simulink model "airbeats"  (R2022a)
settings: Solver=VariableStepAuto  StartTime=0.0  StopTime=10.0  RelTol=1e-3
settings Model: Creator=shobh  LastModifiedBy=shobh

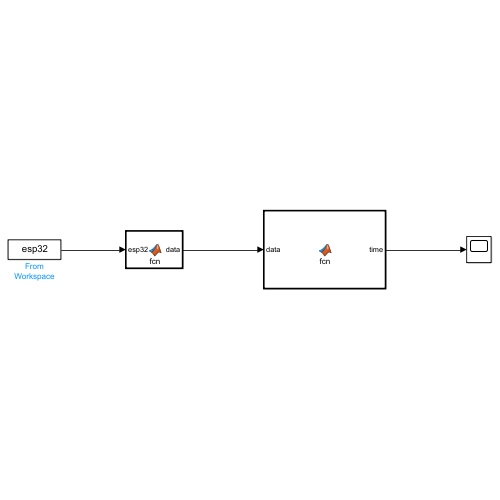
[thumbnail: Simulink's stored preview of the top-level diagram]
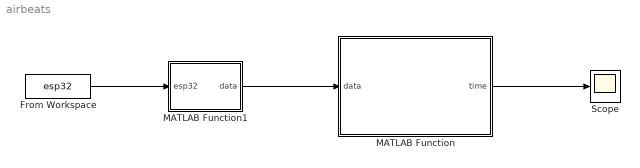
== system airbeats ==
  From Workspace : FromWorkspace  VariableName=esp32
  MATLAB Function : MATLAB Function  TreatAsAtomicUnit=on
  MATLAB Function1 : MATLAB Function  TreatAsAtomicUnit=on
  Scope : Scope
  wires:
  MATLAB Function1/1(data) -> MATLAB Function/1(data)
  MATLAB Function/1(time) -> Scope/1
  From Workspace/1 -> MATLAB Function1/1(esp32)

== matlab function airbeats/MATLAB Function ==
  data: data input; time output
function time = fcn(data)

time = data(1);

== matlab function airbeats/MATLAB Function1 ==
  data: esp32 input; data output
function data = fcn(esp32)

if(esp32.NumBytesAvailable > 0)
    dataRead = esp32.readline();
    data = cell2mat(arrayfun(@str2num,transpose(split(dataRead)),'uni',0));
    data = data(1:10);
end
